simulink library "find6DOFSnell_cl"  (R2018b)
settings: Solver=VariableStepAuto  StartTime=0.0  StopTime=10.0  RelTol=1e-3
undefined symbols (not defined in the file or in its folder): GFC2Bottom, GFC2Side, GFC2Slant
libraries: FindUnitVectorComponents_ul x4, snellDotPosition_ul x4, findEulerAngles_ul x1, findPosition_ul x1, findUnitVectors_ul x1
settings Model: Creator=mcobb  LastModifiedBy=MAE-NCSUCORE

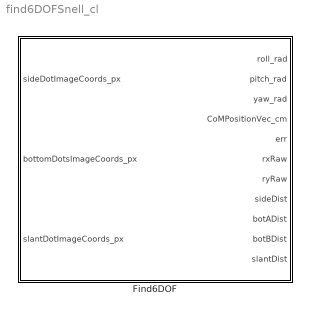
== system find6DOFSnell_cl ==
  Find6DOF : Subsystem  mask{imageDims_px=[1080 2048], initialCoMPositionVec_cm=[0 0 50], cameraFOVAngles_deg=[30 30], sideEulerAngles=[-90 90 0], sideCamPositionVec_cm=[0 0 40], botEulerAngles=[0 0 180], botCamPositionVec_cm=[0 0 0], slantEulerAngles=[180 130 0], slantCamPositionVec_cm=[-20 0 0], sideSeparation_cm=2, sidePositionVecBF_cm=[1 1 1], bottomASeparation_cm=2, botAPositionVecBF_cm=[1 1 1], bottomBSeparation_cm=2, botBPositionVecBG_cm=[1 1 1]}
      mask prompts: imageDims_px "Image Dimensions [rows, cols] [px]"; initialCoMPositionVec_cm "Initial CoM Position Vector [cm]"; cameraFOVAngles_deg "Field of View Angles [horiz, vert] [deg]"; sideEulerAngles "Euler Angles [roll pitch yaw] [deg]"; sideCamPositionVec_cm "Position Vector [cm]"; botEulerAngles "Euler Angles [roll pitch yaw]  [deg]"; botCamPositionVec_cm "Position Vector [cm]"; slantEulerAngles "Euler Angles [roll pitch yaw]  [deg]"; slantCamPositionVec_cm "Position Vec [cm]"; sideSeparation_cm "Separation Distance [cm]"; sidePositionVecBF_cm "Centroid Position in Body Frame [cm]"; bottomASeparation_cm "Separation Distance [cm]"; botAPositionVecBF_cm "Centroid Position in Body Frame [cm]"; bottomBSeparation_cm "Separation Distance [cm]"; botBPositionVecBG_cm "Centroid Position in Body Frame [cm]"
      mask init:
      | find6DOF_init
      mask DialogControl Container4 Prompt: Camera Properties
      mask DialogControl Container14 Prompt: Side Camera
      mask DialogControl Container17 Prompt: Bottom Camera
      mask DialogControl Container18 Prompt: Slant Camera
      mask DialogControl Container13 Prompt: Dot Properties
      mask DialogControl Container11 Prompt: Side Dots
      mask DialogControl Container12 Prompt: Bottom Dot Set A
      mask DialogControl Container15 Prompt: Bottom Dot Set B
      mask Display:
      | image('blockImage.png',[.2, .2, .6, .6],'on');
      | 
      | port_label('input',1,'Side')
      | port_label('input',2,'Bottom')
      | port_label('input',3,'Slant')
      | 
      | port_label('output',1,'roll_rad')
      | port_label('output',2,'pitch_rad')
      | port_label('output',3,'yaw_rad')
      | port_label('output',4,'CoMPosVec_cm')
      | port_label('output',5,'err')
      | 
      | text(0.5, 1, 'Resolve 6 DOF', 'horizontalAlignment', 'center', ...
      |   'verticalAlignment', 'top')

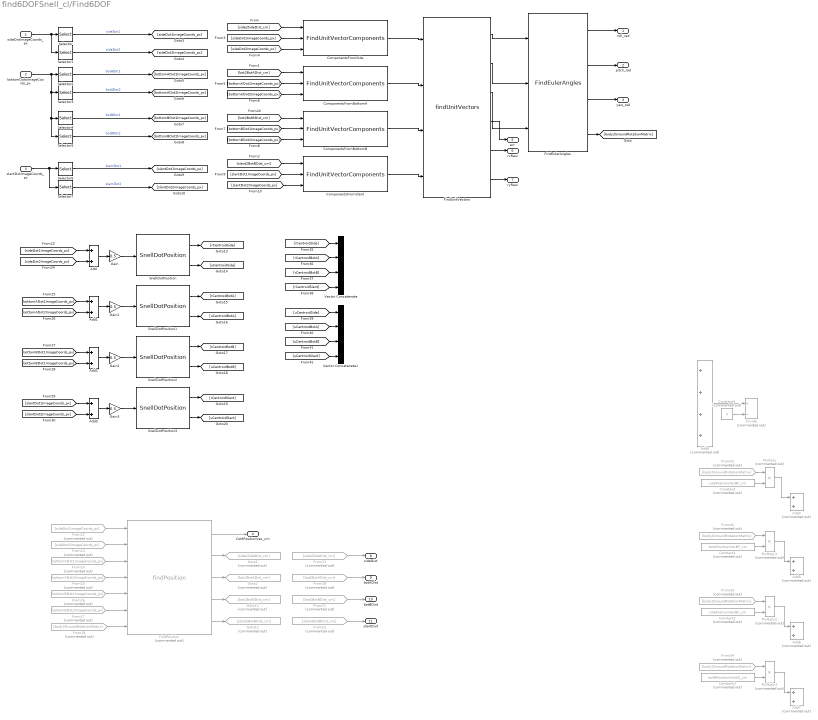
== system find6DOFSnell_cl/Find6DOF ==
  sideDotImageCoords_px : Inport
  bottomDotsImageCoords_px : Inport  Port=2
  slantDotImageCoords_px : Inport  Port=3
  Add{,1..3} (4 alike) : Sum
  Add{4..7} (4 alike) : Sum  Commented=on
  Add8 : Sum  Commented=on  Inputs=++++
  ComponentsFromBottomA : FindUnitVectorComponents_ul/FindUnitVectorComponents  cameraViewAngleVec_deg=cameraFOVAngles_deg  cam2GroundRotationMatrix=GFC2Bottom'  imageDimensions=imageDims_px
  ComponentsFromBottomB : FindUnitVectorComponents_ul/FindUnitVectorComponents  cameraViewAngleVec_deg=cameraFOVAngles_deg  cam2GroundRotationMatrix=GFC2Bottom'  imageDimensions=imageDims_px
  ComponentsFromSide : FindUnitVectorComponents_ul/FindUnitVectorComponents  cameraViewAngleVec_deg=cameraFOVAngles_deg  cam2GroundRotationMatrix=GFC2Side'  imageDimensions=imageDims_px
  ComponentsFromSlant : FindUnitVectorComponents_ul/FindUnitVectorComponents  cameraViewAngleVec_deg=cameraFOVAngles_deg  cam2GroundRotationMatrix=GFC2Slant'  imageDimensions=imageDims_px
  Constant : Constant  Commented=on  Value=sidePositionVecBF_cm
  Constant1 : Constant  Commented=on  Value=botAPositionVecBF_cm
  Constant2 : Constant  Commented=on  Value=sidePositionVecBF_cm
  Constant3 : Constant  Commented=on  Value=botBPositionVecBG_cm
  Constant4 : Constant  Commented=on  Value=4
  Divide : Product  Commented=on  Inputs=*/
  FindEulerAngles : findEulerAngles_ul/FindEulerAngles  SystemSampleTime=-1
  FindPosition : findPosition_ul/findPosition  Commented=on  sideCameraPositionVec_cm=sideCamPositionVec_cm  bottomCameraPositionVec_cm=botCamPositionVec_cm  slantCameraPositionVec_cm=slantCamPositionVec_cm  sideDotPositionVec_cm=sidePositionVecBF_cm  bottomDotAPositionVec_cm=botAPositionVecBF_cm  bottomDotBPositionVec_cm=botBPositionVecBG_cm  side2GroundRotationMatrix=GFC2Side'  bot2GroundRotationMatrix=GFC2Bottom'  slant2GroundRotationMatrix=GFC2Slant'  initialCoMPositionVec_cm=initialCoMPositionVec_cm  imageDims=imageDims_px  cameraFOVAngle_deg=cameraFOVAngles_deg
  FindUnitVectors : findUnitVectors_ul/findUnitVectors  sideSeparation_cm=sideSeparation_cm  bottomASeparation_cm=bottomASeparation_cm  bottomBSeparation_cm=bottomBSeparation_cm  DSB=DSB  DBL=DBL
  From11 : From  Commented=on  GotoTag=side2SideDist_cm
  From12 : From  Commented=on  GotoTag=sideDot1ImageCoords_px
  From13 : From  Commented=on  GotoTag=sideDot2ImageCoords_px
  From14 : From  Commented=on  GotoTag=bottomADot1ImageCoords_px
  From15 : From  Commented=on  GotoTag=bottomADot2ImageCoords_px
  From16 : From  Commented=on  GotoTag=bottomBDot1ImageCoords_px
  From17 : From  Commented=on  GotoTag=bottomBDot2ImageCoords_px
  From18 : From  Commented=on  GotoTag=bot2BotADist_cm
  From{19,31..34} (5 alike) : From  Commented=on  GotoTag=body2GroundRotationMatrix
  From21 : From  Commented=on  GotoTag=bot2BotBDist_cm
  From22 : From  Commented=on  GotoTag=slant2BotBDist_cm
  Gain{,1..3} (4 alike) : Gain  Gain=0.5
  Goto1 : Goto  Commented=on  GotoTag=side2SideDist_cm
  Goto11 : Goto  Commented=on  GotoTag=bot2BotBDist_cm
  Goto12 : Goto  Commented=on  GotoTag=slant2BotBDist_cm
  Goto2 : Goto  Commented=on  GotoTag=bot2BotADist_cm
  Multiply{,1..3} (4 alike) : Product  Commented=on
  Selector : Selector  InputPortWidth=4  IndexOptions=Index vector (dialog)  Indices=[1 2]  OutputSizes=1
  Selector1 : Selector  InputPortWidth=4  IndexOptions=Index vector (dialog)  Indices=[3 4]  OutputSizes=1
  Selector2 : Selector  InputPortWidth=8  IndexOptions=Index vector (dialog)  Indices=[1 2]  OutputSizes=1
  Selector3 : Selector  InputPortWidth=8  IndexOptions=Index vector (dialog)  Indices=[3 4]  OutputSizes=1
  Selector4 : Selector  InputPortWidth=8  IndexOptions=Index vector (dialog)  Indices=[5 6]  OutputSizes=1
  Selector5 : Selector  InputPortWidth=8  IndexOptions=Index vector (dialog)  Indices=[7 8]  OutputSizes=1
  Selector6 : Selector  InputPortWidth=4  IndexOptions=Index vector (dialog)  Indices=[1 2]  OutputSizes=1
  Selector7 : Selector  InputPortWidth=4  IndexOptions=Index vector (dialog)  Indices=[3 4]  OutputSizes=1
  SnellDotPosition : snellDotPosition_ul/SnellDotPosition  camPosVec_cm=sideCamPositionVec_cm  cameraEulerAngles_deg=sideEulerAngles  cameraFOV_deg=cameraFOVAngles_deg  imageDims_px=imageDims_px  dist2Glass=5  indOfRef=[1.000293,1.52,1.333]  glassPlane=xz  glassThickness=2
  SnellDotPosition1 : snellDotPosition_ul/SnellDotPosition  camPosVec_cm=botCamPositionVec_cm  cameraEulerAngles_deg=botEulerAngles  cameraFOV_deg=cameraFOVAngles_deg  imageDims_px=imageDims_px  dist2Glass=5  indOfRef=[1.000293,1.52,1.333]  glassPlane=xy  glassThickness=2
  SnellDotPosition2 : snellDotPosition_ul/SnellDotPosition  camPosVec_cm=botCamPositionVec_cm  cameraEulerAngles_deg=botEulerAngles  cameraFOV_deg=cameraFOVAngles_deg  imageDims_px=imageDims_px  dist2Glass=5  indOfRef=[1.000293,1.52,1.333]  glassPlane=xy  glassThickness=2
  SnellDotPosition3 : snellDotPosition_ul/SnellDotPosition  camPosVec_cm=slantCamPositionVec_cm  cameraEulerAngles_deg=slantEulerAngles  cameraFOV_deg=cameraFOVAngles_deg  imageDims_px=imageDims_px  dist2Glass=5  indOfRef=[1.000293,1.52,1.333]  glassPlane=xy  glassThickness=2
  Vector Concatenate : Concatenate  NumInputs=4  Mode=Multidimensional array  ConcatenateDimension=2
  Vector Concatenate1 : Concatenate  NumInputs=4  Mode=Multidimensional array  ConcatenateDimension=2
  roll_rad : Outport  Unit=rad
  pitch_rad : Outport  Port=2  Unit=rad
  yaw_rad : Outport  Port=3  Unit=rad
  CoMPositionVec_cm : Outport  Port=4  Unit=cm
  err : Outport  Port=5
  rxRaw : Outport  Port=6
  ryRaw : Outport  Port=7
  sideDist : Outport  Port=8
  botADist : Outport  Port=9
  botBDist : Outport  Port=10
  slantDist : Outport  Port=11
  wires:
  ComponentsFromSide/1 -> FindUnitVectors/1
  ComponentsFromBottomA/1 -> FindUnitVectors/2
  ComponentsFromBottomB/1 -> FindUnitVectors/3
  ComponentsFromSlant/1 -> FindUnitVectors/4
  FindUnitVectors/2 -> FindEulerAngles/2
  FindUnitVectors/1 -> FindEulerAngles/1
  FindUnitVectors/3 -> FindEulerAngles/3
  FindPosition/1 -> CoMPositionVec_cm/1
  [sideDot1ImageCoords_px] -> ComponentsFromSide/2
  [sideDot2ImageCoords_px] -> ComponentsFromSide/3
  [bottomADot1ImageCoords_px] -> ComponentsFromBottomA/2
  [bottomADot2ImageCoords_px] -> ComponentsFromBottomA/3
  [bottomBDot1ImageCoords_px] -> ComponentsFromBottomB/2
  [bottomBDot2ImageCoords_px] -> ComponentsFromBottomB/3
  [slantDot1ImageCoords_px] -> ComponentsFromSlant/2
  [slantDot2ImageCoords_px] -> ComponentsFromSlant/3
  FindEulerAngles/1 -> roll_rad/1
  FindEulerAngles/2 -> pitch_rad/1
  FindEulerAngles/3 -> yaw_rad/1
  FindEulerAngles/4 -> [body2GroundRotationMatrix]
  FindUnitVectors/4 -> err/1
  FindPosition/2 -> Goto1/1
  FindPosition/3 -> Goto2/1
  FindPosition/5 -> Goto12/1
  FindPosition/4 -> Goto11/1
  [side2SideDist_cm] -> ComponentsFromSide/1
  [bot2BotADist_cm] -> ComponentsFromBottomA/1
  [slant2BotBDist_cm] -> ComponentsFromSlant/1
  [bot2BotBDist_cm] -> ComponentsFromBottomB/1
  Selector/1 -> [sideDot1ImageCoords_px]  "sideDot1"
  Selector1/1 -> [sideDot2ImageCoords_px]  "sideDot2"
  sideDotImageCoords_px/1 -> Selector1/1, Selector/1
  bottomDotsImageCoords_px/1 -> Selector5/1, Selector4/1, Selector3/1, Selector2/1
  Selector2/1 -> [bottomADot1ImageCoords_px]  "botADot1"
  Selector3/1 -> [bottomADot2ImageCoords_px]  "botADot2"
  Selector4/1 -> [bottomBDot1ImageCoords_px]  "botBDot1"
  Selector5/1 -> [bottomBDot2ImageCoords_px]  "botBDot2"
  Selector6/1 -> [slantDot1ImageCoords_px]  "slantDot1"
  slantDotImageCoords_px/1 -> Selector7/1, Selector6/1
  Selector7/1 -> [slantDot2ImageCoords_px]  "slantDot2"
  From12/1 -> FindPosition/1
  From13/1 -> FindPosition/2
  From14/1 -> FindPosition/3
  From15/1 -> FindPosition/4
  From16/1 -> FindPosition/5
  From17/1 -> FindPosition/6
  From19/1 -> FindPosition/7
  FindUnitVectors/5 -> rxRaw/1
  FindUnitVectors/6 -> ryRaw/1
  From22/1 -> slantDist/1
  From21/1 -> botBDist/1
  From18/1 -> botADist/1
  From11/1 -> sideDist/1
  Add2/1 -> Gain2/1
  Add/1 -> Gain/1
  Add1/1 -> Gain1/1
  Gain/1 -> SnellDotPosition/1
  [sideDot2ImageCoords_px] -> Add/2
  [sideDot1ImageCoords_px] -> Add/1
  [bottomADot1ImageCoords_px] -> Add1/1
  [bottomADot2ImageCoords_px] -> Add1/2
  [bottomBDot1ImageCoords_px] -> Add2/1
  [bottomBDot1ImageCoords_px] -> Add2/2
  [slantDot1ImageCoords_px] -> Add3/1
  [slantDot2ImageCoords_px] -> Add3/2
  Add3/1 -> Gain3/1
  Gain1/1 -> SnellDotPosition1/1
  Gain2/1 -> SnellDotPosition2/1
  Gain3/1 -> SnellDotPosition3/1
  Multiply/1 -> Add4/1
  From31/1 -> Multiply/1
  Constant/1 -> Multiply/2
  From32/1 -> Multiply1/1
  Constant1/1 -> Multiply1/2
  Multiply1/1 -> Add5/1
  Multiply2/1 -> Add6/1
  Constant2/1 -> Multiply2/2
  From33/1 -> Multiply2/1
  Multiply3/1 -> Add7/1
  Constant3/1 -> Multiply3/2
  From34/1 -> Multiply3/1
  Add8/1 -> Divide/1
  Constant4/1 -> Divide/2
  SnellDotPosition/1 -> [rCentroidSide]
  SnellDotPosition/2 -> [uCentroidSide]
  SnellDotPosition1/2 -> [uCentroidBotA]
  SnellDotPosition1/1 -> [rCentroidBotA]
  SnellDotPosition2/2 -> [uCentroidBotB]
  SnellDotPosition2/1 -> [rCentroidBotB]
  SnellDotPosition3/2 -> [uCentroidSlant]
  SnellDotPosition3/1 -> [rCentroidSlant]
  [rCentroidSide] -> Vector Concatenate/1
  [rCentroidBotA] -> Vector Concatenate/2
  [rCentroidBotB] -> Vector Concatenate/3
  [rCentroidSlant] -> Vector Concatenate/4
  [uCentroidSide] -> Vector Concatenate1/1
  [uCentroidBotA] -> Vector Concatenate1/2
  [uCentroidBotB] -> Vector Concatenate1/3
  [uCentroidSlant] -> Vector Concatenate1/4
